simulink model "Vary_RlungNonlinear"  (R2020a)
settings: Solver=VariableStepAuto  StartTime=0.0  StopTime=17  RelTol=1e-3
settings Model: Creator=PrasunOrchi  LastModifiedBy=PrasunOrchi

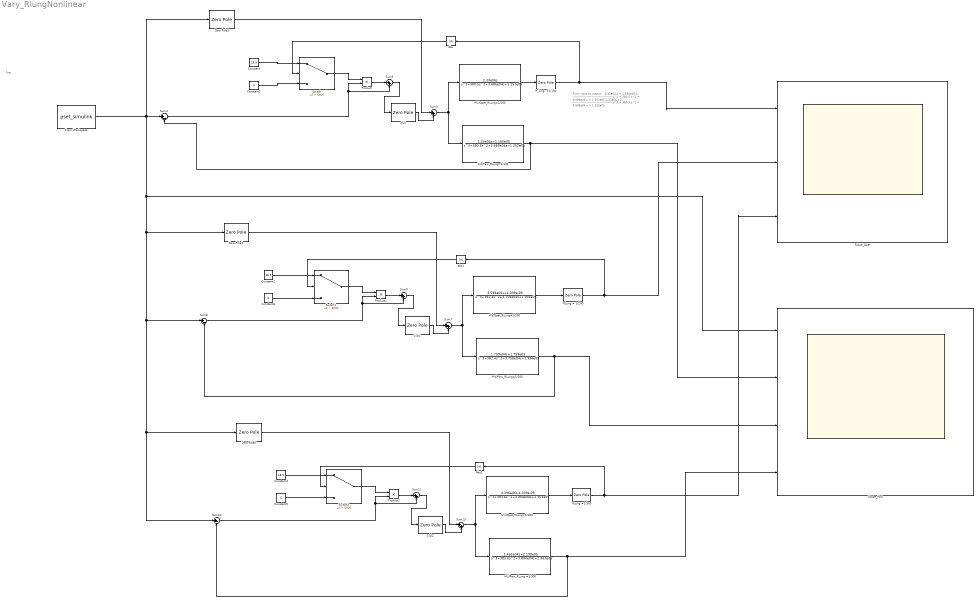
== system Vary_RlungNonlinear ==
  note: From input to output...
      |                 2.33e04 s + 1.165e05
      |    1:  ---------------------------------------
      |        s^3 + 380.5 s^2 + 3.686e04 s + 1.252e05
      |
      |                       2.33e06 s
      |    2:  ---------------------------------------
      |        s^3 + 380.5 s^2 + 3.686e04 s + 1.252e05
  note: Pset
  Abs : Abs
  Abs1 : Abs
  Abs2 : Abs
  C(s) : ZeroPole  Zeros=[]  Poles=[0]  Gain=[0.4]
  C(s)1 : ZeroPole  Zeros=[]  Poles=[0]  Gain=[0.4]
  C(s)2 : ZeroPole  Zeros=[]  Poles=[0]  Gain=[0.4]
  Constant : Constant  Value=18.5
  Constant1 : Constant  Value=0
  Constant2 : Constant  Value=18.5
  Constant3 : Constant  Value=0
  Constant4 : Constant  Value=18.5
  Constant5 : Constant  Value=0
  From Workspace : FromWorkspace  VariableName=pset_simulink
  H(s)Paw_RLung =1/300 : TransferFcn  Numerator=[1.465e04 2.198e05]  Denominator=[1 383.6 3.804e04 2.363e05]
  H(s)Paw_RLung=1/100 : TransferFcn  Numerator=[2.33e04 1.165e05]  Denominator=[1 380.5 3.686e04 1.252e05]
  H(s)Paw_RLung=1/200 : TransferFcn  Numerator=[1.799e04 1.799e05]  Denominator=[1 382.4 3.758e04 1.934e05]
  H(s)Qpat_RLung=1/100 : TransferFcn  Numerator=[2.33e06 0]  Denominator=[1 380.5 3.686e04 1.252e05]
  H(s)Qpat_RLung=1/200 : TransferFcn  Numerator=[3.598e06 4.039e-09]  Denominator=[1 382.4 3.758e04 1.934e05]
  H(s)Qpat_RLung=1/300 : TransferFcn  Numerator=[4.396e06 -4.039e-09]  Denominator=[1 383.6 3.804e04 2.363e05]
  Product : Product
  Product1 : Product
  Product2 : Product
  RLung = 1/200 : ZeroPole  Zeros=[]  Poles=[]  Gain=[60]
  RLung =1/300 : ZeroPole  Zeros=[]  Poles=[]  Gain=[60]
  R_lung  =1/100 : ZeroPole  Zeros=[]  Poles=[]  Gain=[60]
  Scope_Paw : Scope  NumInputPorts=4
  Scope_Qpat : Scope  NumInputPorts=3
  Sum10 : Sum  Inputs=|+-
  Sum{3,5,7,9,11,13} (6 alike) : Sum  Inputs=|++
  Sum4 : Sum  Inputs=|+-
  Sum8 : Sum  Inputs=|+-
  Switch : Switch  Criteria=u2 > Threshold  Threshold=6000
  Switch1 : Switch  Criteria=u2 > Threshold  Threshold=6000
  Switch2 : Switch  Criteria=u2 > Threshold  Threshold=6000
  Zero-Pole1 : ZeroPole  Zeros=[]  Poles=[]
  Zero-Pole3 : ZeroPole  Zeros=[]  Poles=[]
  Zero-Pole5 : ZeroPole  Zeros=[]  Poles=[]
  wires:
  Abs2/1 -> Switch2/2
  Product2/1 -> Sum11/1
  Zero-Pole5/1 -> Sum13/1
  Sum13/1 -> H(s)Qpat_RLung=1/300/1, H(s)Paw_RLung =1/300/1
  C(s)1/1 -> Sum7/2
  Sum8/1 -> Sum9/2, Product1/2
  Sum9/1 -> C(s)1/1
  Switch/1 -> Product/1
  Sum11/1 -> C(s)2/1
  Abs/1 -> Switch/2
  Constant3/1 -> Switch1/3
  H(s)Qpat_RLung=1/100/1 -> R_lung  =1/100/1
  Switch2/1 -> Product2/1
  R_lung  =1/100/1 -> Abs/1, Scope_Qpat/1
  RLung = 1/200/1 -> Abs1/1, Scope_Qpat/2
  C(s)2/1 -> Sum13/2
  Sum7/1 -> H(s)Qpat_RLung=1/200/1, H(s)Paw_RLung=1/200/1
  Switch1/1 -> Product1/1
  Constant1/1 -> Switch/3
  Sum3/1 -> H(s)Qpat_RLung=1/100/1, H(s)Paw_RLung=1/100/1
  Sum5/1 -> C(s)/1
  Product1/1 -> Sum9/1
  Constant2/1 -> Switch1/1
  Sum4/1 -> Sum5/2, Product/2
  H(s)Paw_RLung =1/300/1 -> Sum10/2, Scope_Paw/4
  H(s)Qpat_RLung=1/300/1 -> RLung =1/300/1
  From Workspace/1 -> Sum4/1, Zero-Pole1/1, Scope_Paw/1, Zero-Pole3/1, Zero-Pole5/1, Sum10/1, Sum8/1
  Zero-Pole1/1 -> Sum3/1
  H(s)Paw_RLung=1/100/1 -> Scope_Paw/2, Sum4/2
  Product/1 -> Sum5/1
  Constant/1 -> Switch/1
  H(s)Paw_RLung=1/200/1 -> Sum8/2, Scope_Paw/3
  Abs1/1 -> Switch1/2
  RLung =1/300/1 -> Abs2/1, Scope_Qpat/3
  Constant4/1 -> Switch2/1
  Sum10/1 -> Sum11/2, Product2/2
  C(s)/1 -> Sum3/2
  Constant5/1 -> Switch2/3
  H(s)Qpat_RLung=1/200/1 -> RLung = 1/200/1
  Zero-Pole3/1 -> Sum7/1
